simulink model "ServerSimulink"  (R2024a)
settings: Solver=VariableStepAuto  StartTime=0.0  StopTime=10.0  RelTol=1e-3
libraries: fuzblock x1
settings Model: Creator=Admin  LastModifiedBy=Admin

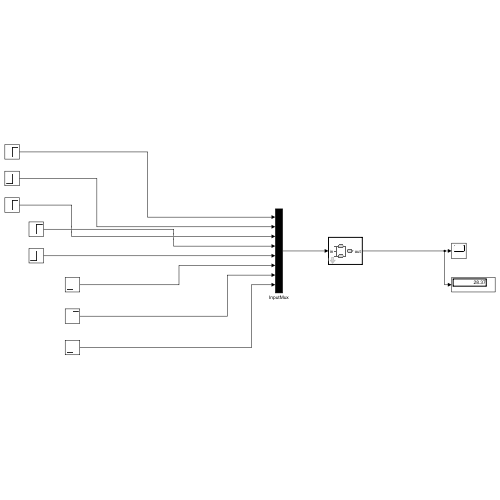
[thumbnail: Simulink's stored preview of the top-level diagram]
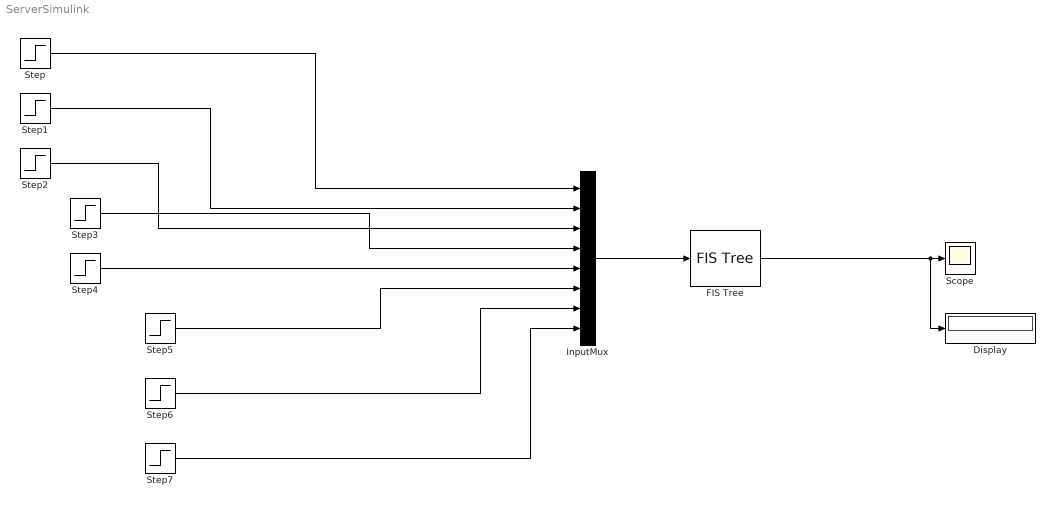
== system ServerSimulink ==
  Display : Display
  FIS Tree : fuzblock/FIS Tree  FIS=ServerFailureModel  OutputSampleNumber=101  DataType=double  SimulateUsing=Interpreted execution  OutOfRangeInputValueMessage=warning  NoRuleFiredMessage=warning  EmptyOutputFuzzySetMessage=warning
  InputMux : Mux  Inputs=8
  Scope : Scope
  Step : Step  After=20  SampleTime=0
  Step1 : Step  After=55  SampleTime=0
  Step2 : Step  After=5  SampleTime=0
  Step3 : Step  After=3  SampleTime=0
  Step4 : Step  After=7  SampleTime=0
  Step5 : Step  After=2  SampleTime=0
  Step6 : Step  After=30  SampleTime=0
  Step7 : Step  After=8  SampleTime=0
  wires:
  FIS Tree/1 -> Display/1, Scope/1
  InputMux/1 -> FIS Tree/1
  Step/1 -> InputMux/1
  Step1/1 -> InputMux/2
  Step2/1 -> InputMux/3
  Step3/1 -> InputMux/4
  Step4/1 -> InputMux/5
  Step5/1 -> InputMux/6
  Step6/1 -> InputMux/7
  Step7/1 -> InputMux/8
